simulink model "CompleteAttDetSim"  (R2018b)
settings: Solver=FixedStepAuto  StartTime=0.0  StopTime=24*3600  FixedStep=10  RelTol=1e-3  EnableMultiTasking=on
PreLoadFcn:
  | InitialiseJ2
values from neighbouring files (symbols this model uses):
  AngMomentum = (grav_parameter*rp*(1 + eccentricity))^0.5    [InitialiseJ2.m]
  Arg_periapsis = D3(1,6)    [InitialiseJ2.m]
  earthRadius = 6378.137    [InitialiseJ2.m]
  eccentricity = D3(1,5)/1e7    [InitialiseJ2.m]
  grav_parameter = 398600.4415    [InitialiseJ2.m]
  inclination = D3(1,3)    [InitialiseJ2.m]
  J2 = 0.0010836    [InitialiseJ2.m]
  period = 2*pi*sqrt(sm_axis^3/grav_parameter)    [InitialiseJ2.m]
  RAAN = D3(1,4)    [InitialiseJ2.m]
  sm_axis = (grav_parameter/(avg_motion*2*pi/(24*3600))^2)^(1/3)    [InitialiseJ2.m]
  t0 = avg_anomaly/(2*pi)*period    [InitialiseJ2.m]
undefined symbols (not defined in the file or in its folder): Earth, WGS84
libraries: vrlib x11, sharedtransform x7, simulink x6, aerolibutil x4, aerolibtransform2 x1
(part 1 of 2)
settings Model: PauseTimes=0  NumberOfSteps=10  SnapshotBufferSize=10000  SnapshotInterval=1  Creator="TEAM  STUDSAT -2"  LastModifiedBy=lauren
settings OptimizationCC: LifeSpan=inf
settings DebuggingCC: SFUnexpectedBacktrackingDiag=warning  SFNoUnconditionalDefaultTransitionDiag=warning  SFExecutionAtInitializationDiag=none
settings SFSimCC: SimUseLocalCustomCode=off
settings RTWCC: RTWUseLocalCustomCode=off
settings CodeAppCC: StateflowObjectComments=on
settings GRTTargetCC: TargetLangStandard=C89/C90 (ANSI)  GeneratePreprocessorConditionals=Disable all
settings ConfigComp: CovMetricSettings=dw  CovHtmlReporting=on  CovSaveCumulativeToWorkspaceVar=on  CovSaveSingleToWorkspaceVar=on  CovExternalEMLEnable=off
settings SimscapeCC: SimscapeNormalizeSystem=off

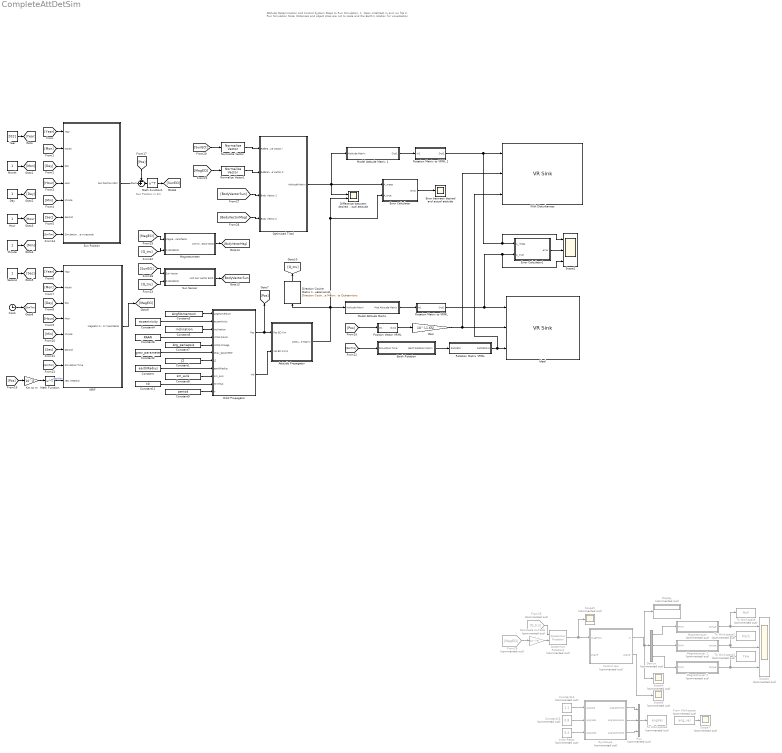
== system CompleteAttDetSim ==
  note: Sun Position in Km
  note: Attitude Determination and Control System
      |
      | Steps to Run Simulation:
      | 1. Open initalizeJ2.m and run file
      | 2. Run Simulation
      |
      | Note:
      | Distances and object sizes are not to scale and the Earth's rotation for visualisation
  " Magnetometer" : Subsystem
  " Sun Position" : Subsystem
  Attitude Propagator : Subsystem
  Clock : Clock
  Constant : Constant  Value=earthRadius
  Constant1 : Constant  Value=J2
  Constant11 : Constant  Value=t0
  Constant14 : Constant  Commented=on  Value=1.1
  Constant15 : Constant  Commented=on  Value=0.8
  Constant2 : Constant  Value=grav_parameter
  Constant3 : Constant  Value=AngMomentum
  Constant4 : Constant  Value=eccentricity
  Constant5 : Constant  Value=inclination
  Constant6 : Constant  Value=RAAN
  Constant7 : Constant  Value=Arg_periapsis
  Constant8 : Constant  Value=sm_axis
  Constant9 : Constant  Value=period
  Control Law : MATLAB Function  Commented=on  TreatAsAtomicUnit=on
  Day : Constant
  Demux : Demux  Commented=on  Outputs=3
  Difference between desired and actual attitude : Scope  NumInputPorts=2
  Direction Cosine Matrix to Quaternions1 : sharedtransform/Direction Cosine Matrix  to Quaternions  aMode=aMode  action=None  tolerance=eps(2)
      settings: SourceProductName=Aerospace Blockset  SourceProductBaseCode=AE
  Display : Display  Commented=on
  Earth Rotation : Subsystem
  Error Calculator : Subsystem
  Error Calculator1 : Subsystem
  Error between desired and actual attitude : Scope
  From Workspace : FromWorkspace  Commented=on  VariableName=ang_vel  SampleTime=0
  From28 : From  Commented=on  GotoTag=MagECI
  From29 : From  Commented=on  GotoTag=Q_tru
  Gain : Gain  Gain=10^(-1.65)
  Gyroscope : Subsystem  Commented=on
  Hour : Constant
  IGRF : Subsystem
  Ideal : vrlib/VR Sink  InstantiateOnLoad=on  SampleTime=-1  ViewEnable=on  RemoteChange=off  RemoteView=off  FieldsWritten=Satellite.rotation.4.1.1.double#Satellite.translation.3.1.1.double#Earth.rotation.4.1.1.double  WorldFileName=earthSatSys_Ideal.WRL  AutoView=off  VideoDimensions=[]  AllowVariableSize=off
      settings: SourceProductBaseCode=VR
  "Initial Rates " : Constant  Commented=on  Value=0.4
  Km to m : Gain  Gain=10^3
  "Magnetorquer " : Subsystem  Commented=on
  Magnetorquer 1 : Subsystem  Commented=on
  Magnetorquer 2 : Subsystem  Commented=on
  Math Function : Math  Operator=transpose  SaturateOnIntegerOverflow=on
  Math Function1 : Math  Operator=transpose  SaturateOnIntegerOverflow=on
  Minute : Constant
  Model Attitude Martix : Subsystem
  Model Attitude Matrix 1 : Subsystem
  Month : Constant
  Mux : Mux  Commented=on  Inputs=3
  Nanotesla to Tesla : Gain  Commented=on  Gain=10^(-9)
  Normalize Vector : vrlib/Utilities/Normalize Vector  maxzero=0
      settings: SourceProductName=Simulink 3D Animation  SourceProductBaseCode=VR
  Normalize Vector1 : vrlib/Utilities/Normalize Vector  maxzero=0
      settings: SourceProductName=Simulink 3D Animation  SourceProductBaseCode=VR
  Optimised Triad : Subsystem
  Orbit Propagator : Subsystem
  Position Vector VRML : Subsystem
  Quaternion Rotation1 : aerolibutil/Quaternion Rotation  Commented=on
  Rotation Matrix VRML : Subsystem
  "Rotation Matrix to VRML " : Subsystem
  Rotation Matrix to VRML 1 : Subsystem
  Scope1 : Scope  NumInputPorts=3
  Scope2 : Scope  Commented=on  NumInputPorts=3
  Scope{4..7} (4 alike) : Scope  Commented=on
  Second : Constant
  Sum : Sum  Inputs=-+|
  Sun Sensor : Subsystem
  To Workspace : ToWorkspace  Commented=on  VariableName=Roll  SampleTime=-1
  To Workspace1 : ToWorkspace  Commented=on  VariableName=Yaw  SampleTime=-1
  To Workspace2 : ToWorkspace  Commented=on  VariableName=Pitch  SampleTime=-1
  To Workspace3 : ToWorkspace  Commented=on  VariableName=angVel  SaveFormat=Timeseries  SampleTime=-1
  With Disturbances : vrlib/VR Sink  InstantiateOnLoad=on  SampleTime=-1  ViewEnable=on  RemoteChange=off  RemoteView=off  FieldsWritten=Satellite1.rotation.4.1.1.double#Satellite1.translation.3.1.1.double#Earth1.rotation.4.1.1.double  WorldFileName=earthSatSys_Real.WRL  AutoView=off  VideoDimensions=[]  AllowVariableSize=off
      settings: SourceProductBaseCode=VR
  Year : Constant  Value=2021
  wires:
  Constant/1 -> Orbit Propagator/8(earthRadius)
  Constant1/1 -> Orbit Propagator/7(J2)
  Constant2/1 -> Orbit Propagator/6(Grav_parameter)
  Constant3/1 -> Orbit Propagator/1(angMomentum)
  Constant4/1 -> Orbit Propagator/2(eccentricity)
  Constant5/1 -> Orbit Propagator/3(inclination)
  Constant6/1 -> Orbit Propagator/4(initial RAAN)
  Constant8/1 -> Orbit Propagator/9(sm_axis)
  Constant11/1 -> Orbit Propagator/10(t0 initial)
  Constant9/1 -> Orbit Propagator/11(T)
  Constant7/1 -> Orbit Propagator/5(initial Omega)
  Earth Rotation/1(Earth Rotation Matrix) -> Rotation Matrix VRML/1(RotMatIn)
  Position Vector VRML/1(Out1) -> Gain/1
  Gain/1 -> With Disturbances/2, Ideal/2
  Model Attitude Martix/1(Mod Attitude Matrix) -> "Rotation Matrix to VRML "/1(In1)
  Orbit Propagator/2(Vel) -> Attitude Propagator/2(Vel ECI Km/s)
  "Rotation Matrix to VRML "/1(Out1) -> Ideal/1, Scope1/3, Error Calculator1/2(A_true)
  Model Attitude Matrix 1/1(Out1) -> Rotation Matrix to VRML 1/1(In1)
  Rotation Matrix to VRML 1/1(Out1) -> Scope1/1, Error Calculator1/1(A_meas), With Disturbances/1
  Km to m/1 -> Math Function/1
  " Sun Position"/1(Sun Position (ECI)) -> Sum/2
  Year/1 -> [Year]
  Month/1 -> [Mon]
  Day/1 -> [Day]
  Hour/1 -> [Hour]
  Minute/1 -> [Min]
  Second/1 -> [Sec]
  [Year] -> " Sun Position"/1(Year)
  [Mon] -> " Sun Position"/2("Month ")
  [Day] -> " Sun Position"/3(Day)
  [Hour] -> " Sun Position"/4(Hour)
  [Min] -> " Sun Position"/5(Minute)
  [Sec] -> " Sun Position"/6(Second)
  [Year] -> IGRF/1(Year)
  [Mon] -> IGRF/2(Month)
  [Day] -> IGRF/3(Day)
  [Hour] -> IGRF/4(Hour)
  [Min] -> IGRF/5(Minute)
  [Sec] -> IGRF/6(Second)
  Clock/1 -> [SimTim]
  [SimTim] -> Earth Rotation/1(Simulation Time)
  [SimTim] -> IGRF/7(Simulation Time)
  [SimTim] -> " Sun Position"/7(Simulation time in seconds)
  Orbit Propagator/1(Pos) -> Attitude Propagator/1(Pos ECI Km), [Pos]
  [Pos] -> Position Vector VRML/1(In1)
  [Pos] -> Km to m/1
  Math Function/1 -> IGRF/8(rECI (Meters))  "position"
  [Pos] -> Sum/1
  Sum/1 -> Math Function1/1
  IGRF/1(Magnetic Field in ECI (nanoTesla)) -> [MagECI]
  [SunECI] -> Sun Sensor/1(Sun Vector)
  [MagECI] -> " Magnetometer"/1(Magnettic Field ECI nanoTesla)
  [SunECI] -> Normalize Vector/1
  [MagECI] -> Normalize Vector1/1
  Normalize Vector/1 -> Optimised Triad/1(Reference Vector !)
  Normalize Vector1/1 -> Optimised Triad/2(Reference Vector 2)
  Direction Cosine Matrix to Quaternions1/1 -> [Q_tru]
  [Q_tru] -> " Magnetometer"/2(Q ECI2BOD)
  [Q_tru] -> Sun Sensor/2(Q ECI2BOD)
  Math Function1/1 -> [SunECI]
  Optimised Triad/1(Attitude Matrix) -> Difference between desired and actual attitude/1, Error Calculator/1(A_meas), Model Attitude Matrix 1/1(Attitude Matrix)
  Attitude Propagator/1(Attitude Matrix) -> Model Attitude Martix/1(Attitude Matrix), Error Calculator/2(A_true), Difference between desired and actual attitude/2, Direction Cosine Matrix to Quaternions1/1
  Sun Sensor/1(Unit Sun Vector BOD) -> [BodyVectorSun]
  [BodyVectorSun] -> Optimised Triad/3(Body Vector 1)
  [BodyVectorMag] -> Optimised Triad/4(Body Vector 2)
  Error Calculator1/1(error) -> Scope1/2
  Error Calculator/1(error) -> Error between desired and actual attitude/1
  Rotation Matrix VRML/1(RotMatOut) -> With Disturbances/3, Ideal/3
  " Magnetometer"/1(Unit Magnetic Field Vector BOD) -> [BodyVectorMag]
  Gyroscope/1(angratenoise) -> Mux/1
  Gyroscope/2("angratenoise1 ") -> Mux/2
  Gyroscope/3("angratenoise2 ") -> Mux/3
  Demux/1 -> "Magnetorquer "/1(PWM)
  Demux/2 -> Magnetorquer 1/1("PWM ")
  Demux/3 -> Magnetorquer 2/1(PWM)
  Magnetorquer 1/1(torque) -> Scope2/2, To Workspace2/1
  "Magnetorquer "/1(torque) -> Scope2/1, To Workspace/1
  Magnetorquer 2/1(torque) -> Scope2/3, To Workspace1/1
  Control Law/1(m) -> Scope4/1, Display/1, Demux/1
  Nanotesla to Tesla/1 -> Quaternion Rotation1/2
  From28/1 -> Nanotesla to Tesla/1
  From29/1 -> Quaternion Rotation1/1
  Quaternion Rotation1/1 -> Scope5/1, Control Law/1(magField)
  Control Law/2(angvel) -> Scope6/1
  Constant14/1 -> Gyroscope/1(angrate)
  Constant15/1 -> Gyroscope/2("angrate1 ")
  "Initial Rates "/1 -> Gyroscope/3(angrate2)
  Mux/1 -> To Workspace3/1
  From Workspace/1 -> Scope7/1

== system CompleteAttDetSim/ Magnetometer ==
  Magnettic Field ECI nanoTesla : Inport
  Q ECI2BOD : Inport  Port=2
  Magnetometer Error : Subsystem
  Nanotesla to Tesla : Gain  Gain=10^(-9)
  Normalize Vector5 : vrlib/Utilities/Normalize Vector  maxzero=0
      settings: SourceProductName=Simulink 3D Animation  SourceProductBaseCode=VR
  Quaternion Rotation1 : aerolibutil/Quaternion Rotation
  Unit Magnetic Field Vector BOD : Outport
  wires:
  Magnettic Field ECI nanoTesla/1 -> Nanotesla to Tesla/1
  Magnetometer Error/1("Magnetic Field BOD (Tesla)1 ") -> Normalize Vector5/1
  Normalize Vector5/1 -> Unit Magnetic Field Vector BOD/1
  Q ECI2BOD/1 -> Quaternion Rotation1/1
  Nanotesla to Tesla/1 -> Quaternion Rotation1/2
  Quaternion Rotation1/1 -> Magnetometer Error/1(Magnetic Field BOD (Tesla))

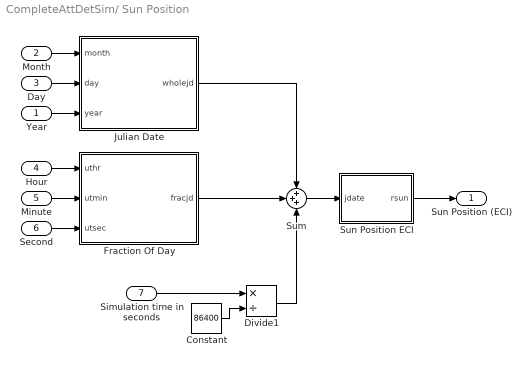
== system CompleteAttDetSim/ Sun Position ==
  Year : Inport
  "Month " : Inport  Port=2
  Day : Inport  Port=3
  Hour : Inport  Port=4
  Minute : Inport  Port=5
  Second : Inport  Port=6
  Simulation time in seconds : Inport  Port=7
  Constant : Constant  Value=86400
  Divide1 : Product  Inputs=*/
  Fraction Of Day : MATLAB Function  TreatAsAtomicUnit=on
  Julian Date : MATLAB Function  TreatAsAtomicUnit=on
  Sum : Sum  Inputs=+++
  Sun Position ECI : MATLAB Function  TreatAsAtomicUnit=on
  Sun Position (ECI) : Outport
  wires:
  Sum/1 -> Sun Position ECI/1(jdate)
  Simulation time in seconds/1 -> Divide1/1
  Sun Position ECI/1(rsun) -> Sun Position (ECI)/1
  Second/1 -> Fraction Of Day/3(utsec)
  Fraction Of Day/1(fracjd) -> Sum/2
  Year/1 -> Julian Date/3(year)
  Day/1 -> Julian Date/2(day)
  Divide1/1 -> Sum/3
  Minute/1 -> Fraction Of Day/2(utmin)
  Julian Date/1(wholejd) -> Sum/1
  Constant/1 -> Divide1/2
  Hour/1 -> Fraction Of Day/1(uthr)
  "Month "/1 -> Julian Date/1(month)

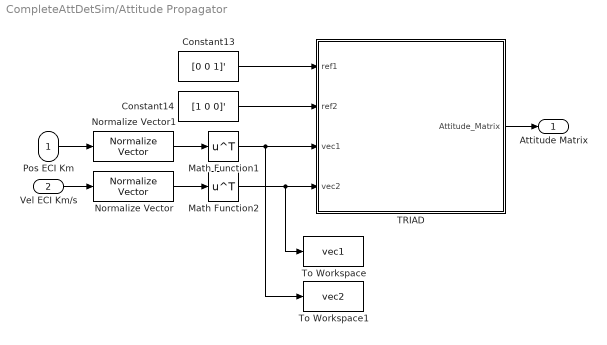
== system CompleteAttDetSim/Attitude Propagator ==
  Pos ECI Km : Inport
  Vel ECI Km/s : Inport  Port=2
  Constant13 : Constant  Value=[0 0 1]'  VectorParams1D=off
  Constant14 : Constant  Value=[1 0 0]'  VectorParams1D=off
  Math Function1 : Math  Operator=transpose  SaturateOnIntegerOverflow=on
  Math Function2 : Math  Operator=transpose  SaturateOnIntegerOverflow=on
  Normalize Vector : vrlib/Utilities/Normalize Vector  maxzero=0
      settings: SourceProductName=Simulink 3D Animation  SourceProductBaseCode=VR
  Normalize Vector1 : vrlib/Utilities/Normalize Vector  maxzero=0
      settings: SourceProductName=Simulink 3D Animation  SourceProductBaseCode=VR
  TRIAD : MATLAB Function  TreatAsAtomicUnit=on
  To Workspace : ToWorkspace  VariableName=vec1  SampleTime=-1
  To Workspace1 : ToWorkspace  VariableName=vec2  SampleTime=-1
  Attitude Matrix : Outport
  wires:
  Constant13/1 -> TRIAD/1(ref1)
  TRIAD/1(Attitude_Matrix) -> Attitude Matrix/1
  Math Function1/1 -> To Workspace1/1, TRIAD/3(vec1)
  Math Function2/1 -> To Workspace/1, TRIAD/4(vec2)
  Constant14/1 -> TRIAD/2(ref2)
  Vel ECI Km/s/1 -> Normalize Vector/1
  Normalize Vector/1 -> Math Function2/1
  Normalize Vector1/1 -> Math Function1/1
  Pos ECI Km/1 -> Normalize Vector1/1

== system CompleteAttDetSim/Earth Rotation ==
  Simulation Time : Inport
  Constant10 : Constant  Value=0.004178074378280
  Subsystem1 : Subsystem
  Earth Rotation Matrix : Outport
  wires:
  Constant10/1 -> Subsystem1/1(we)
  Simulation Time/1 -> Subsystem1/2(Clock)
  Subsystem1/1(Earth Rotation Matrix) -> Earth Rotation Matrix/1

== system CompleteAttDetSim/Error Calculator ==
  A_meas : Inport
  A_true : Inport  Port=2
  Subtract : Sum  Inputs=+-
  error : Outport
  wires:
  Subtract/1 -> error/1
  A_meas/1 -> Subtract/1
  A_true/1 -> Subtract/2

== system CompleteAttDetSim/Error Calculator1 ==
  A_meas : Inport
  A_true : Inport  Port=2
  Subtract : Sum  Inputs=+-
  error : Outport
  wires:
  Subtract/1 -> error/1
  A_meas/1 -> Subtract/1
  A_true/1 -> Subtract/2

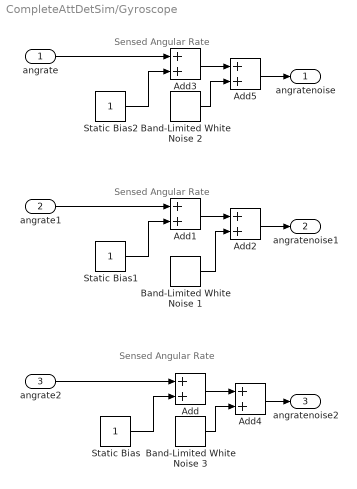
== system CompleteAttDetSim/Gyroscope ==
  note: Sensed Angular Rate
  note: Sensed Angular Rate
  note: Sensed Angular Rate
  angrate : Inport
  "angrate1 " : Inport  Port=2
  angrate2 : Inport  Port=3
  Add{,1..5} (6 alike) : Sum
  Band-Limited White Noise 1 : simulink/Sources/Band-Limited White Noise  Cov=[0.018^2]  Ts=10  seed=[23341]
  Band-Limited White Noise 2 : simulink/Sources/Band-Limited White Noise  Cov=[0.018^2]  Ts=10  seed=[23341]
  Band-Limited White Noise 3 : simulink/Sources/Band-Limited White Noise  Cov=[0.018^2]  Ts=10  seed=[23341]
  Static Bias : Constant
  Static Bias1 : Constant
  Static Bias2 : Constant
  angratenoise : Outport
  "angratenoise1 " : Outport  Port=2
  "angratenoise2 " : Outport  Port=3
  wires:
  Add4/1 -> "angratenoise2 "/1
  Add2/1 -> "angratenoise1 "/1
  Add5/1 -> angratenoise/1
  Band-Limited White Noise 3/1 -> Add4/2
  Static Bias/1 -> Add/2
  Add/1 -> Add4/1
  angrate2/1 -> Add/1
  Static Bias1/1 -> Add1/2
  Add1/1 -> Add2/1
  Band-Limited White Noise 1/1 -> Add2/2
  "angrate1 "/1 -> Add1/1
  Static Bias2/1 -> Add3/2
  Add3/1 -> Add5/1
  Band-Limited White Noise 2/1 -> Add5/2
  angrate/1 -> Add3/1

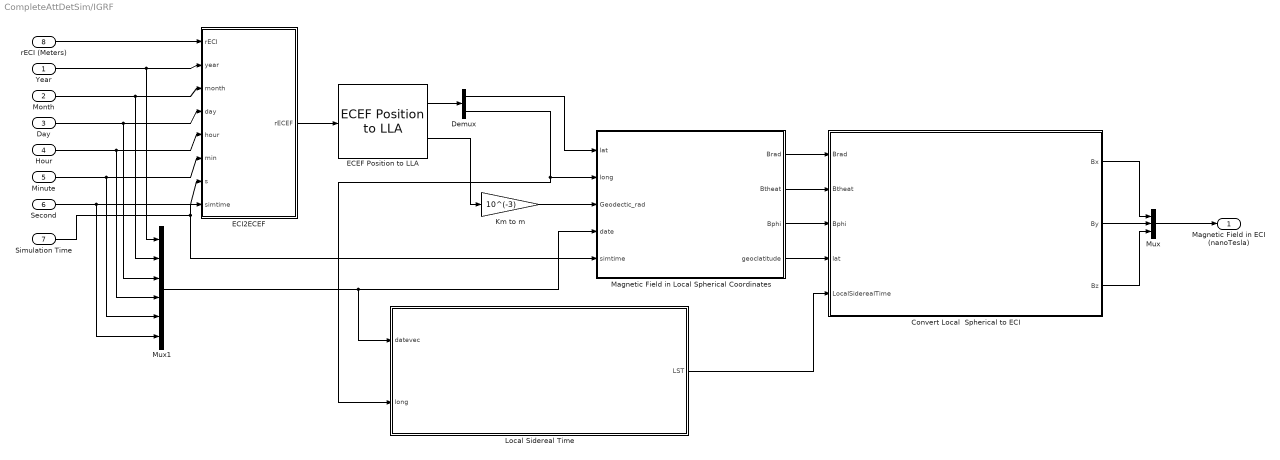
== system CompleteAttDetSim/IGRF ==
  Year : Inport
  Month : Inport  Port=2
  Day : Inport  Port=3
  Hour : Inport  Port=4
  Minute : Inport  Port=5
  Second : Inport  Port=6
  Simulation Time : Inport  Port=7
  rECI (Meters) : Inport  Port=8
  Convert Local  Spherical to ECI : MATLAB Function  TreatAsAtomicUnit=on
  Demux : Demux  Outputs=2
  ECEF Position to LLA : aerolibtransform2/ECEF Position to LLA  units=Metric (MKS)  ptype=Earth (WGS84)  F=1/298.257223563  R=6378137
      settings: SourceProductName=Aerospace Blockset  SourceProductBaseCode=AE
  ECI2ECEF : MATLAB Function  TreatAsAtomicUnit=on
  Km to m : Gain  Gain=10^(-3)
  Local Sidereal Time : MATLAB Function  TreatAsAtomicUnit=on
  Magnetic Field in Local Spherical Coordinates : MATLAB Function  TreatAsAtomicUnit=on
  Mux : Mux  Inputs=3
  Mux1 : Mux  Inputs=6
  Magnetic Field in ECI (nanoTesla) : Outport
  wires:
  Magnetic Field in Local Spherical Coordinates/2(Btheat) -> Convert Local  Spherical to ECI/2(Btheat)
  Day/1 -> Mux1/3, ECI2ECEF/4(day)
  Second/1 -> Mux1/6, ECI2ECEF/7(s)
  ECEF Position to LLA/1 -> Demux/1
  Convert Local  Spherical to ECI/3(Bz) -> Mux/3
  Magnetic Field in Local Spherical Coordinates/3(Bphi) -> Convert Local  Spherical to ECI/3(Bphi)
  Local Sidereal Time/1(LST) -> Convert Local  Spherical to ECI/5(LocalSiderealTime)
  Magnetic Field in Local Spherical Coordinates/1(Brad) -> Convert Local  Spherical to ECI/1(Brad)
  ECEF Position to LLA/2 -> Km to m/1
  Minute/1 -> Mux1/5, ECI2ECEF/6(min)
  ECI2ECEF/1(rECEF) -> ECEF Position to LLA/1
  Demux/1 -> Magnetic Field in Local Spherical Coordinates/1(lat)
  Month/1 -> Mux1/2, ECI2ECEF/3(month)
  Year/1 -> Mux1/1, ECI2ECEF/2(year)
  rECI (Meters)/1 -> ECI2ECEF/1(rECI)
  Convert Local  Spherical to ECI/1(Bx) -> Mux/1
  Magnetic Field in Local Spherical Coordinates/4(geoclatitude) -> Convert Local  Spherical to ECI/4(lat)
  Hour/1 -> Mux1/4, ECI2ECEF/5(hour)
  Mux1/1 -> Magnetic Field in Local Spherical Coordinates/4(date), Local Sidereal Time/1(datevec)
  Convert Local  Spherical to ECI/2(By) -> Mux/2
  Demux/2 -> Local Sidereal Time/2(long), Magnetic Field in Local Spherical Coordinates/2(long)
  Mux/1 -> Magnetic Field in ECI (nanoTesla)/1
  Simulation Time/1 -> ECI2ECEF/8(simtime), Magnetic Field in Local Spherical Coordinates/5(simtime)
  Km to m/1 -> Magnetic Field in Local Spherical Coordinates/3(Geodectic_rad)

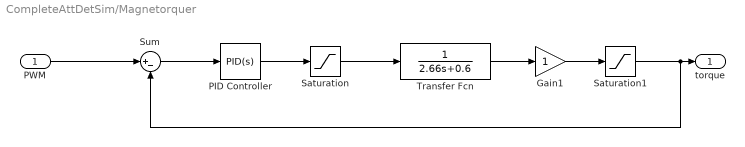
== system CompleteAttDetSim/Magnetorquer  ==
  PWM : Inport
  Gain1 : Gain
  PID Controller : simulink/Continuous/PID Controller  Controller=PID  Form=Parallel  TimeDomain=Continuous-time  SampleTime=-1  IntegratorMethod=Forward Euler  FilterMethod=Forward Euler  ControllerParametersSource=internal  P=3  I=1  D=0  UseFilter=on  N=100  TunerSelectOption=Transfer Function Based (PID Tuner App)  InitialConditionSource=internal  InitialConditionForIntegrator=0  InitialConditionForFilter=0  DifferentiatorICPrevScaledInput=0  ExternalReset=none  TrackingMode=off  Kt=1  LimitOutput=off  UpperSaturationLimit=inf  LowerSaturationLimit=-inf  LinearizeAsGain=on  AntiWindupMode=none  Kb=1  POutMin=[]  POutMax=[]  IOutMin=[]  IOutMax=[]  DOutMin=[]  DOutMax=[]  NOutMin=[]  NOutMax=[]  SumOutMin=[]  SumOutMax=[]  SaturationOutMin=[]  SaturationOutMax=[]  PParamMin=[]  PParamMax=[]  IParamMin=[]  IParamMax=[]  DParamMin=[]  DParamMax=[]  NParamMin=[]  NParamMax=[]  KbParamMin=[]  KbParamMax=[]  KtParamMin=[]  KtParamMax=[]  KbOutMin=[]  KbOutMax=[]  KtOutMin=[]  KtOutMax=[]  IntegratorOutMin=[]  IntegratorOutMax=[]  FilterOutMin=[]  FilterOutMax=[]  SumI1OutMin=[]  SumI1OutMax=[]  SumI2OutMin=[]  SumI2OutMax=[]  SumI3OutMin=[]  SumI3OutMax=[]  SumI4OutMin=[]  SumI4OutMax=[]  SumDOutMin=[]  SumDOutMax=[]  DifferentiatorOutMin=[]  DifferentiatorOutMax=[]  FilterDiffOutCoefMin=[]  FilterDiffOutCoefMax=[]  ReciprocalOutMin=[]  ReciprocalOutMax=[]  SumDenOutMin=[]  SumDenOutMax=[]  SumNumOutMin=[]  SumNumOutMax=[]  DivideOutMin=[]  DivideOutMax=[]  IntegratorContinuousStateAttributes=''  IntegratorStateMustResolveToSignalObject=off  IntegratorRTWStateStorageClass=Auto  FilterContinuousStateAttributes=''  FilterStateMustResolveToSignalObject=off  FilterRTWStateStorageClass=Auto  ParallelPVariant=InternalParameters  IdealPVariant=Disabled  IVariant=InternalParameters  DVariant=InternalParameters  IntegratorVariant=Continuous  SatVariant=Disabled  AWVariant=Passthrough  PCopyVariant=Disabled  TRVariant=Disabled  FdbkBlocksVariant=Forward  IdealPFdbkVariant=Disabled  SatFdbkVariant=Disabled  DerivativeFilterVariant=ContFilter  NVariant=InternalParameters  NCopyVariant=Disabled  FilterICVariant=InternalICsFilter  IntegratorICVariant=InternalICs  ExternalResetVariant=Disabled  TRSumVariant=Passthrough  SumFdbkVariant=Disabled  SumVariant=Sum_PID
  Saturation : Saturate
  Saturation1 : Saturate
  Sum : Sum  Inputs=|+-
  Transfer Fcn : TransferFcn  Denominator=[2.66 0.6]
  torque : Outport
  wires:
  Gain1/1 -> Saturation1/1
  PID Controller/1 -> Saturation/1
  Transfer Fcn/1 -> Gain1/1
  PWM/1 -> Sum/1
  Sum/1 -> PID Controller/1
  Saturation/1 -> Transfer Fcn/1
  Saturation1/1 -> Sum/2, torque/1

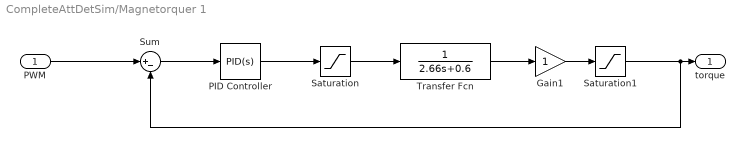
== system CompleteAttDetSim/Magnetorquer 1 ==
  "PWM " : Inport
  Gain1 : Gain
  PID Controller : simulink/Continuous/PID Controller  Controller=PID  Form=Parallel  TimeDomain=Continuous-time  SampleTime=-1  IntegratorMethod=Forward Euler  FilterMethod=Forward Euler  ControllerParametersSource=internal  P=3  I=1  D=0  UseFilter=on  N=100  TunerSelectOption=Transfer Function Based (PID Tuner App)  InitialConditionSource=internal  InitialConditionForIntegrator=0  InitialConditionForFilter=0  DifferentiatorICPrevScaledInput=0  ExternalReset=none  TrackingMode=off  Kt=1  LimitOutput=off  UpperSaturationLimit=inf  LowerSaturationLimit=-inf  LinearizeAsGain=on  AntiWindupMode=none  Kb=1  POutMin=[]  POutMax=[]  IOutMin=[]  IOutMax=[]  DOutMin=[]  DOutMax=[]  NOutMin=[]  NOutMax=[]  SumOutMin=[]  SumOutMax=[]  SaturationOutMin=[]  SaturationOutMax=[]  PParamMin=[]  PParamMax=[]  IParamMin=[]  IParamMax=[]  DParamMin=[]  DParamMax=[]  NParamMin=[]  NParamMax=[]  KbParamMin=[]  KbParamMax=[]  KtParamMin=[]  KtParamMax=[]  KbOutMin=[]  KbOutMax=[]  KtOutMin=[]  KtOutMax=[]  IntegratorOutMin=[]  IntegratorOutMax=[]  FilterOutMin=[]  FilterOutMax=[]  SumI1OutMin=[]  SumI1OutMax=[]  SumI2OutMin=[]  SumI2OutMax=[]  SumI3OutMin=[]  SumI3OutMax=[]  SumI4OutMin=[]  SumI4OutMax=[]  SumDOutMin=[]  SumDOutMax=[]  DifferentiatorOutMin=[]  DifferentiatorOutMax=[]  FilterDiffOutCoefMin=[]  FilterDiffOutCoefMax=[]  ReciprocalOutMin=[]  ReciprocalOutMax=[]  SumDenOutMin=[]  SumDenOutMax=[]  SumNumOutMin=[]  SumNumOutMax=[]  DivideOutMin=[]  DivideOutMax=[]  IntegratorContinuousStateAttributes=''  IntegratorStateMustResolveToSignalObject=off  IntegratorRTWStateStorageClass=Auto  FilterContinuousStateAttributes=''  FilterStateMustResolveToSignalObject=off  FilterRTWStateStorageClass=Auto  ParallelPVariant=InternalParameters  IdealPVariant=Disabled  IVariant=InternalParameters  DVariant=InternalParameters  IntegratorVariant=Continuous  SatVariant=Disabled  AWVariant=Passthrough  PCopyVariant=Disabled  TRVariant=Disabled  FdbkBlocksVariant=Forward  IdealPFdbkVariant=Disabled  SatFdbkVariant=Disabled  DerivativeFilterVariant=ContFilter  NVariant=InternalParameters  NCopyVariant=Disabled  FilterICVariant=InternalICsFilter  IntegratorICVariant=InternalICs  ExternalResetVariant=Disabled  TRSumVariant=Passthrough  SumFdbkVariant=Disabled  SumVariant=Sum_PID
  Saturation : Saturate
  Saturation1 : Saturate
  Sum : Sum  Inputs=|+-
  Transfer Fcn : TransferFcn  Denominator=[2.66 0.6]
  torque : Outport
  wires:
  Gain1/1 -> Saturation1/1
  PID Controller/1 -> Saturation/1
  Transfer Fcn/1 -> Gain1/1
  "PWM "/1 -> Sum/1
  Sum/1 -> PID Controller/1
  Saturation/1 -> Transfer Fcn/1
  Saturation1/1 -> Sum/2, torque/1

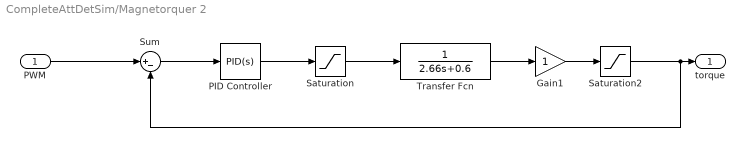
== system CompleteAttDetSim/Magnetorquer 2 ==
  PWM : Inport
  Gain1 : Gain
  PID Controller : simulink/Continuous/PID Controller  Controller=PID  Form=Parallel  TimeDomain=Continuous-time  SampleTime=-1  IntegratorMethod=Forward Euler  FilterMethod=Forward Euler  ControllerParametersSource=internal  P=3  I=1  D=0  UseFilter=on  N=100  TunerSelectOption=Transfer Function Based (PID Tuner App)  InitialConditionSource=internal  InitialConditionForIntegrator=0  InitialConditionForFilter=0  DifferentiatorICPrevScaledInput=0  ExternalReset=none  TrackingMode=off  Kt=1  LimitOutput=off  UpperSaturationLimit=inf  LowerSaturationLimit=-inf  LinearizeAsGain=on  AntiWindupMode=none  Kb=1  POutMin=[]  POutMax=[]  IOutMin=[]  IOutMax=[]  DOutMin=[]  DOutMax=[]  NOutMin=[]  NOutMax=[]  SumOutMin=[]  SumOutMax=[]  SaturationOutMin=[]  SaturationOutMax=[]  PParamMin=[]  PParamMax=[]  IParamMin=[]  IParamMax=[]  DParamMin=[]  DParamMax=[]  NParamMin=[]  NParamMax=[]  KbParamMin=[]  KbParamMax=[]  KtParamMin=[]  KtParamMax=[]  KbOutMin=[]  KbOutMax=[]  KtOutMin=[]  KtOutMax=[]  IntegratorOutMin=[]  IntegratorOutMax=[]  FilterOutMin=[]  FilterOutMax=[]  SumI1OutMin=[]  SumI1OutMax=[]  SumI2OutMin=[]  SumI2OutMax=[]  SumI3OutMin=[]  SumI3OutMax=[]  SumI4OutMin=[]  SumI4OutMax=[]  SumDOutMin=[]  SumDOutMax=[]  DifferentiatorOutMin=[]  DifferentiatorOutMax=[]  FilterDiffOutCoefMin=[]  FilterDiffOutCoefMax=[]  ReciprocalOutMin=[]  ReciprocalOutMax=[]  SumDenOutMin=[]  SumDenOutMax=[]  SumNumOutMin=[]  SumNumOutMax=[]  DivideOutMin=[]  DivideOutMax=[]  IntegratorContinuousStateAttributes=''  IntegratorStateMustResolveToSignalObject=off  IntegratorRTWStateStorageClass=Auto  FilterContinuousStateAttributes=''  FilterStateMustResolveToSignalObject=off  FilterRTWStateStorageClass=Auto  ParallelPVariant=InternalParameters  IdealPVariant=Disabled  IVariant=InternalParameters  DVariant=InternalParameters  IntegratorVariant=Continuous  SatVariant=Disabled  AWVariant=Passthrough  PCopyVariant=Disabled  TRVariant=Disabled  FdbkBlocksVariant=Forward  IdealPFdbkVariant=Disabled  SatFdbkVariant=Disabled  DerivativeFilterVariant=ContFilter  NVariant=InternalParameters  NCopyVariant=Disabled  FilterICVariant=InternalICsFilter  IntegratorICVariant=InternalICs  ExternalResetVariant=Disabled  TRSumVariant=Passthrough  SumFdbkVariant=Disabled  SumVariant=Sum_PID
  Saturation : Saturate
  Saturation2 : Saturate
  Sum : Sum  Inputs=|+-
  Transfer Fcn : TransferFcn  Denominator=[2.66 0.6]
  torque : Outport
  wires:
  Gain1/1 -> Saturation2/1
  PID Controller/1 -> Saturation/1
  Transfer Fcn/1 -> Gain1/1
  PWM/1 -> Sum/1
  Sum/1 -> PID Controller/1
  Saturation/1 -> Transfer Fcn/1
  Saturation2/1 -> Sum/2, torque/1

== system CompleteAttDetSim/Model Attitude Martix ==
  Attitude Matrix : Inport
  Constant10 : Constant  Value=-90
  Matrix Multiply1 : Product  Multiplication=Matrix(*)
  Rotate about x1 : MATLAB Function  TreatAsAtomicUnit=on
  Mod Attitude Matrix : Outport
  wires:
  Constant10/1 -> Rotate about x1/1(u)
  Matrix Multiply1/1 -> Mod Attitude Matrix/1
  Attitude Matrix/1 -> Matrix Multiply1/1
  Rotate about x1/1(y) -> Matrix Multiply1/2

== system CompleteAttDetSim/Model Attitude Matrix 1 ==
  Attitude Matrix : Inport
  Constant10 : Constant  Value=-90
  Matrix Multiply1 : Product  Multiplication=Matrix(*)
  Rotate about x1 : MATLAB Function  TreatAsAtomicUnit=on
  Out1 : Outport
  wires:
  Constant10/1 -> Rotate about x1/1(u)
  Matrix Multiply1/1 -> Out1/1
  Attitude Matrix/1 -> Matrix Multiply1/1
  Rotate about x1/1(y) -> Matrix Multiply1/2

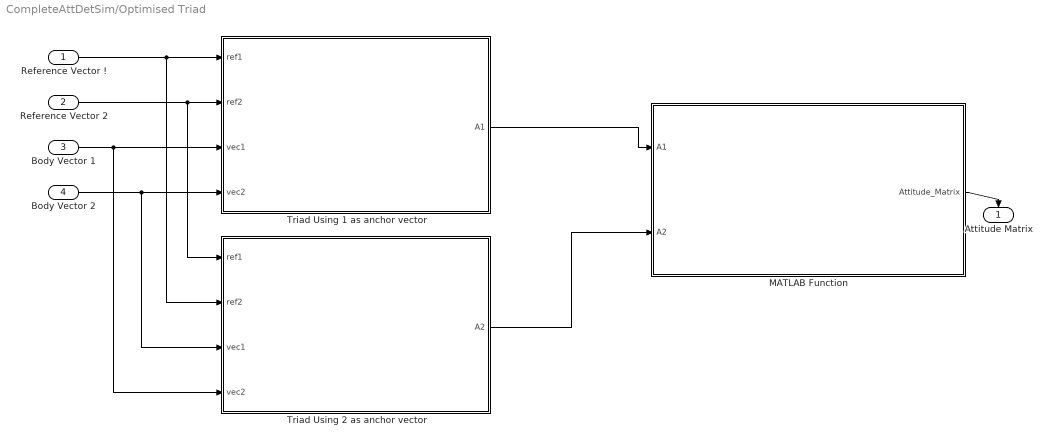
== system CompleteAttDetSim/Optimised Triad ==
  Reference Vector ! : Inport
  Reference Vector 2 : Inport  Port=2
  Body Vector 1 : Inport  Port=3
  Body Vector 2 : Inport  Port=4
  MATLAB Function : MATLAB Function  TreatAsAtomicUnit=on
  Triad Using 1 as anchor vector : MATLAB Function  TreatAsAtomicUnit=on
  Triad Using 2 as anchor vector : MATLAB Function  TreatAsAtomicUnit=on
  Attitude Matrix : Outport
  wires:
  Triad Using 1 as anchor vector/1(A1) -> MATLAB Function/1(A1)
  Body Vector 2/1 -> Triad Using 1 as anchor vector/4(vec2), Triad Using 2 as anchor vector/3(vec1)
  Body Vector 1/1 -> Triad Using 2 as anchor vector/4(vec2), Triad Using 1 as anchor vector/3(vec1)
  Triad Using 2 as anchor vector/1(A2) -> MATLAB Function/2(A2)
  Reference Vector 2/1 -> Triad Using 1 as anchor vector/2(ref2), Triad Using 2 as anchor vector/1(ref1)
  MATLAB Function/1(Attitude_Matrix) -> Attitude Matrix/1
  Reference Vector !/1 -> Triad Using 2 as anchor vector/2(ref2), Triad Using 1 as anchor vector/1(ref1)

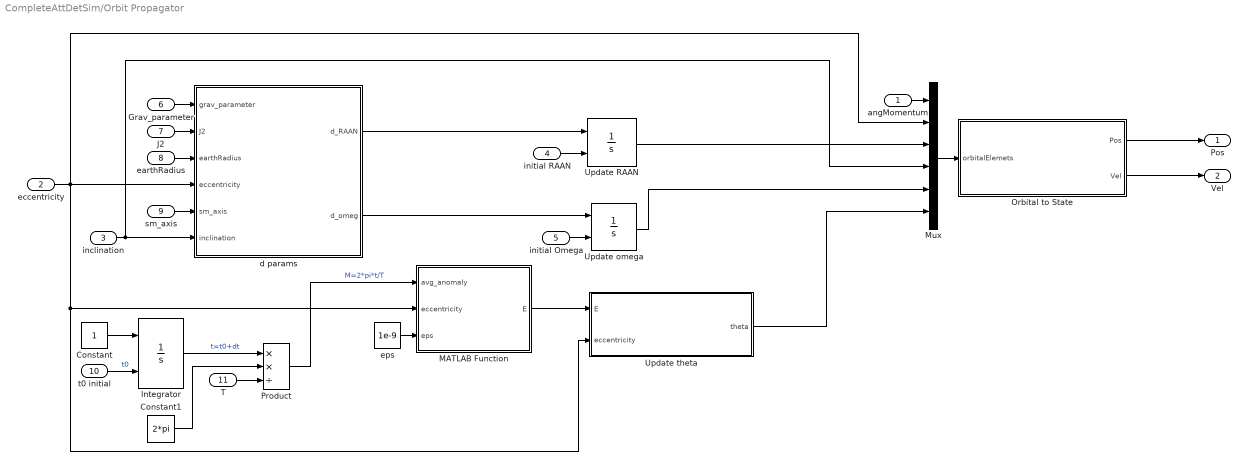
== system CompleteAttDetSim/Orbit Propagator ==
  angMomentum : Inport
  eccentricity : Inport  Port=2
  inclination : Inport  Port=3
  initial RAAN : Inport  Port=4
  initial Omega : Inport  Port=5
  Grav_parameter : Inport  Port=6
  J2 : Inport  Port=7
  earthRadius : Inport  Port=8
  sm_axis : Inport  Port=9
  t0 initial : Inport  Port=10
  T : Inport  Port=11
  Constant : Constant
  Constant1 : Constant  Value=2*pi
  Integrator : Integrator  InitialConditionSource=external
  MATLAB Function : MATLAB Function  TreatAsAtomicUnit=on
  Mux : Mux  Inputs=6
  Orbital to State : MATLAB Function  TreatAsAtomicUnit=on
  Product : Product  Inputs=**/
  Update RAAN : Integrator  InitialConditionSource=external
  Update omega : Integrator  InitialConditionSource=external
  Update theta : MATLAB Function  TreatAsAtomicUnit=on
  d params : MATLAB Function  TreatAsAtomicUnit=on
  eps : Constant  Value=1e-9
  Pos : Outport
  Vel : Outport  Port=2
  wires:
  eps/1 -> MATLAB Function/3(eps)
  Grav_parameter/1 -> d params/1(grav_parameter)
  sm_axis/1 -> d params/5(sm_axis)
  J2/1 -> d params/2(J2)
  earthRadius/1 -> d params/3(earthRadius)
  MATLAB Function/1(E) -> Update theta/1(E)
  t0 initial/1 -> Integrator/2  "t0"
  Constant/1 -> Integrator/1
  Integrator/1 -> Product/1  "t=t0+dt"
  T/1 -> Product/3
  Constant1/1 -> Product/2
  d params/1(d_RAAN) -> Update RAAN/1
  initial RAAN/1 -> Update RAAN/2
  d params/2(d_omeg) -> Update omega/1
  initial Omega/1 -> Update omega/2
  angMomentum/1 -> Mux/1
  inclination/1 -> Mux/4, d params/6(inclination)
  Mux/1 -> Orbital to State/1(orbitalElemets)
  Product/1 -> MATLAB Function/1(avg_anomaly)  "M=2*pi*t/T"
  Update omega/1 -> Mux/5
  Update theta/1(theta) -> Mux/6
  Update RAAN/1 -> Mux/3
  eccentricity/1 -> Update theta/2(eccentricity), MATLAB Function/2(eccentricity), Mux/2, d params/4(eccentricity)
  Orbital to State/1(Pos) -> Pos/1
  Orbital to State/2(Vel) -> Vel/1

== system CompleteAttDetSim/Position Vector VRML ==
  In1 : Inport
  Demux : Demux  Outputs=3
  Gain2 : Gain  Gain=-1
  Mux : Mux  Inputs=3
  Out1 : Outport
  wires:
  Demux/1 -> Mux/1
  Demux/2 -> Gain2/1
  Demux/3 -> Mux/2
  Mux/1 -> Out1/1
  Gain2/1 -> Mux/3
  In1/1 -> Demux/1

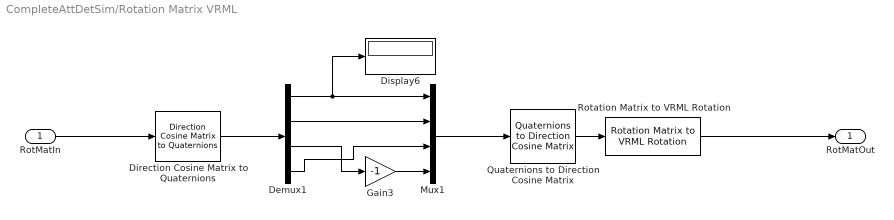
== system CompleteAttDetSim/Rotation Matrix VRML ==
  RotMatIn : Inport
  Demux1 : Demux
  Direction Cosine Matrix to Quaternions : sharedtransform/Direction Cosine Matrix  to Quaternions  aMode=aMode  action=None  tolerance=eps(2)
      settings: SourceProductName=Aerospace Blockset  SourceProductBaseCode=AE
  Display6 : Display
  Gain3 : Gain  Gain=-1
  Mux1 : Mux
  Quaternions to Direction Cosine Matrix : sharedtransform/Quaternions to  Direction Cosine Matrix  aMode=aMode
      settings: SourceProductName=Aerospace Blockset  SourceProductBaseCode=AE
  Rotation Matrix to VRML Rotation : vrlib/Utilities/Rotation Matrix to VRML Rotation  maxzero=1e-12
      settings: SourceProductName=Simulink 3D Animation  SourceProductBaseCode=VR
  RotMatOut : Outport
  wires:
  RotMatIn/1 -> Direction Cosine Matrix to Quaternions/1
  Direction Cosine Matrix to Quaternions/1 -> Demux1/1
  Demux1/3 -> Gain3/1
  Gain3/1 -> Mux1/4
  Demux1/4 -> Mux1/3
  Demux1/2 -> Mux1/2
  Demux1/1 -> Display6/1, Mux1/1
  Mux1/1 -> Quaternions to Direction Cosine Matrix/1
  Quaternions to Direction Cosine Matrix/1 -> Rotation Matrix to VRML Rotation/1
  Rotation Matrix to VRML Rotation/1 -> RotMatOut/1

== system CompleteAttDetSim/Rotation Matrix to VRML  ==
  In1 : Inport
  Demux2 : Demux
  Direction Cosine Matrix to Quaternions1 : sharedtransform/Direction Cosine Matrix  to Quaternions  aMode=aMode  action=None  tolerance=eps(2)
      settings: SourceProductName=Aerospace Blockset  SourceProductBaseCode=AE
  Gain4 : Gain  Gain=-1
  Mux2 : Mux
  Quaternions to Direction Cosine Matrix1 : sharedtransform/Quaternions to  Direction Cosine Matrix  aMode=aMode
      settings: SourceProductName=Aerospace Blockset  SourceProductBaseCode=AE
  Rotation Matrix to VRML Rotation1 : vrlib/Utilities/Rotation Matrix to VRML Rotation  maxzero=1e-12
      settings: SourceProductName=Simulink 3D Animation  SourceProductBaseCode=VR
  Out1 : Outport
  wires:
  Direction Cosine Matrix to Quaternions1/1 -> Demux2/1
  Rotation Matrix to VRML Rotation1/1 -> Out1/1
  Mux2/1 -> Quaternions to Direction Cosine Matrix1/1
  Demux2/4 -> Mux2/3
  Demux2/3 -> Gain4/1
  Gain4/1 -> Mux2/4
  Demux2/1 -> Mux2/1
  Demux2/2 -> Mux2/2
  Quaternions to Direction Cosine Matrix1/1 -> Rotation Matrix to VRML Rotation1/1
  In1/1 -> Direction Cosine Matrix to Quaternions1/1

== system CompleteAttDetSim/Rotation Matrix to VRML 1 ==
  In1 : Inport
  Demux2 : Demux
  Direction Cosine Matrix to Quaternions1 : sharedtransform/Direction Cosine Matrix  to Quaternions  aMode=aMode  action=None  tolerance=eps(2)
      settings: SourceProductName=Aerospace Blockset  SourceProductBaseCode=AE
  Gain4 : Gain  Gain=-1
  Mux2 : Mux
  Quaternions to Direction Cosine Matrix1 : sharedtransform/Quaternions to  Direction Cosine Matrix  aMode=aMode
      settings: SourceProductName=Aerospace Blockset  SourceProductBaseCode=AE
  Rotation Matrix to VRML Rotation1 : vrlib/Utilities/Rotation Matrix to VRML Rotation  maxzero=1e-12
      settings: SourceProductName=Simulink 3D Animation  SourceProductBaseCode=VR
  Out1 : Outport
  wires:
  Direction Cosine Matrix to Quaternions1/1 -> Demux2/1
  Rotation Matrix to VRML Rotation1/1 -> Out1/1
  Mux2/1 -> Quaternions to Direction Cosine Matrix1/1
  Demux2/4 -> Mux2/3
  Demux2/3 -> Gain4/1
  Gain4/1 -> Mux2/4
  Demux2/1 -> Mux2/1
  Demux2/2 -> Mux2/2
  Quaternions to Direction Cosine Matrix1/1 -> Rotation Matrix to VRML Rotation1/1
  In1/1 -> Direction Cosine Matrix to Quaternions1/1

== system CompleteAttDetSim/Sun Sensor ==
  Sun Vector : Inport
  Q ECI2BOD : Inport  Port=2
  Normalize Vector4 : vrlib/Utilities/Normalize Vector  maxzero=0
      settings: SourceProductName=Simulink 3D Animation  SourceProductBaseCode=VR
  Quaternion Rotation : aerolibutil/Quaternion Rotation
  Quaternion Rotation2 : aerolibutil/Quaternion Rotation
  Random Quat Error : MATLAB Function  TreatAsAtomicUnit=on
  Unit Sun Vector BOD : Outport
  wires:
  Sun Vector/1 -> Quaternion Rotation/2
  Random Quat Error/1(quat) -> Quaternion Rotation/1
  Normalize Vector4/1 -> Unit Sun Vector BOD/1
  Q ECI2BOD/1 -> Quaternion Rotation2/1
  Quaternion Rotation2/1 -> Normalize Vector4/1
  Quaternion Rotation/1 -> Quaternion Rotation2/2

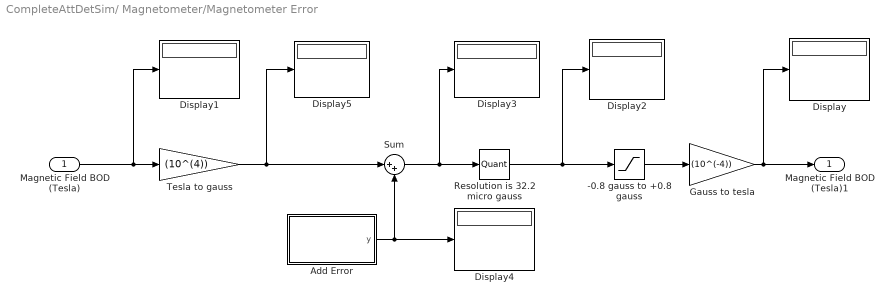
== system CompleteAttDetSim/ Magnetometer/Magnetometer Error ==
  Magnetic Field BOD (Tesla) : Inport
  -0.8 gauss to +0.8 gauss : Saturate  UpperLimit=0.8  LowerLimit=-0.8
  Add Error : MATLAB Function  TreatAsAtomicUnit=on
  Display{,1..5} (6 alike) : Display
  Gauss to tesla : Gain  Gain=(10^(-4))
  Resolution is 32.2 micro gauss : Quantizer  QuantizationInterval=0.0322
  Sum : Sum  Inputs=|++
  Tesla to gauss : Gain  Gain=(10^(4))
  "Magnetic Field BOD (Tesla)1 " : Outport
  wires:
  -0.8 gauss to +0.8 gauss/1 -> Gauss to tesla/1
  Sum/1 -> Display3/1, Resolution is 32.2 micro gauss/1
  Tesla to gauss/1 -> Sum/1, Display5/1
  Add Error/1(y) -> Display4/1, Sum/2
  Magnetic Field BOD (Tesla)/1 -> Display1/1, Tesla to gauss/1
  Gauss to tesla/1 -> "Magnetic Field BOD (Tesla)1 "/1, Display/1
  Resolution is 32.2 micro gauss/1 -> -0.8 gauss to +0.8 gauss/1, Display2/1

== system CompleteAttDetSim/Earth Rotation/Subsystem1 ==
  we : Inport
  Clock : Inport  Port=2
  Display : Display
  MATLAB Function : MATLAB Function  TreatAsAtomicUnit=on
  Product1 : Product
  Earth Rotation Matrix : Outport
  wires:
  Clock/1 -> Product1/2
  we/1 -> Product1/1
  Product1/1 -> MATLAB Function/1(u), Display/1  "fi_earth"
  MATLAB Function/1(y) -> Earth Rotation Matrix/1

== matlab function CompleteAttDetSim/Earth Rotation/Subsystem1/MATLAB Function ==
  data: u input; y output
function y = fcn(u)
y =rotz(u);

== matlab function CompleteAttDetSim/Orbit Propagator/d params ==
  data: grav_parameter input; d_RAAN output; J2 input; earthRadius input; eccentricity input; sm_axis input; inclination input; d_omeg output
function [d_RAAN, d_omeg]=dparams(grav_parameter,J2, earthRadius,eccentricity,sm_axis,inclination)
d_RAAN = -(1.5*J2*grav_parameter^0.5*earthRadius^2/((1-eccentricity^2)*sm_axis^3.5))*cosd(inclination)*180/pi;
d_omeg = d_RAAN*(2.5*sind(inclination)^2 - 2)/cosd(inclination);
end

== matlab function CompleteAttDetSim/Model Attitude Matrix 1/Rotate about x1 ==
  data: u input; y output
function y = fcn(u)
y =rotx(u);

== matlab function CompleteAttDetSim/Orbit Propagator/MATLAB Function ==
  data: avg_anomaly input; eccentricity input; E output; eps input
function E = keplerEq(avg_anomaly,eccentricity,eps)
En  = avg_anomaly;
Ens = En - (En-eccentricity*sin(En)- avg_anomaly)/...
    (1 - eccentricity*cos(En));
while ( abs(Ens-En) > eps )
    En = Ens;
    Ens = En - (En - eccentricity*sin(En) - avg_anomaly)/...
        (1 - eccentricity*cos(En));
end
E = Ens;
end

== matlab function CompleteAttDetSim/Orbit Propagator/Update theta ==
  data: E input; theta output; eccentricity input
function theta = updateTheta(E,eccentricity)
theta=2*atan(tan(E/2)*((1+eccentricity)/(1-eccentricity))^0.5)*180/pi;
end

== matlab function CompleteAttDetSim/Orbit Propagator/Orbital to State ==
  data: orbitalElemets input; Pos output size=[1 3]; Vel output size=[1 3]
function [Pos, Vel] = Orbital2State(orbitalElemets)

% ˜˜˜˜˜˜˜˜˜˜˜˜˜˜˜˜˜˜˜˜˜˜˜˜˜˜˜˜˜˜˜˜˜˜
% This function computes the state vector (r,v) from the
% classical orbital elements (coe).
%
% 
% incl = inclination of the orbit (rad)
% w = argument of perigee (rad)
% TA = true anomaly (rad)
% R3_w - Rotation matrix about the z-axis through the angle w
% R1_i - Rotation matrix about the x-axis through the angle i
% Rot_z - Rotation matrix about the z-axis through the angle RA
% Q_pX - Matrix of the transformation from perifocal to
% geocentric equatorial frame

% r - position vector in the geocentric equatorial frame
% (km)
% v - velocity vector in the geocentric equatorial frame
% (km/s)
%
% User M-functions required: none
% ------------------------------------------------------------
grav_parameter = 398600; 
angMomentum = orbitalElemets(1);
eccentricity = orbitalElemets(2);
RAAN = orbitalElemets(3)*pi/180;
inclination = orbitalElemets(4)*pi/180;
omega = orbitalElemets(5)*pi/180;
theta = orbitalElemets(6)*pi/180;

%perifocal_frame_posVect - position vector in the perifocal frame in kilometers
% perifocal_frame_velVect - velocity vector in the perifocal frame in kilometers per second
perifocal_frame_posVect =(angMomentum^2/grav_parameter)*(1/(1+eccentricity*cos(theta)))*(cos(theta)*[1;0;0]+ sin(theta)*[0;1;0]);
perifocal_frame_velVect =(grav_parameter/angMomentum)*(-sin(theta)*[1;0;0]+(eccentricity+cos(theta))*[0;1;0]);

%Rotation matrix about z-axis through angle RAAN
Rot_zw = [ cos(RAAN) sin(RAAN) 0; -sin(RAAN) cos(RAAN) 0; 0 0 1];
%Rotation matrix about x-axis through the angle of inclination
Rot_xi = [1 0 0; 0 cos(inclination) sin(inclination); 0 -sin(inclination) cos(inclination)];
%Rotation matrix about the z-axis through the angle omega
R3_w = [ cos(omega) sin(omega) 0; -sin(omega) cos(omega) 0; 0 0 1];
%transformation from perifocal to geocentric equatorial frame
Geo_to_equatorial = Rot_zw'*Rot_xi'*R3_w';
% position and velocity vector in the geocentric equatorial frame in kilometers per second
pos = Geo_to_equatorial*perifocal_frame_posVect;
vel = Geo_to_equatorial*perifocal_frame_velVect;

Pos = pos';
Vel = vel';
% ˜˜˜˜˜˜˜˜˜˜˜˜˜˜˜˜˜˜˜˜˜˜˜˜˜˜˜˜˜˜˜˜˜˜˜˜˜˜˜˜˜˜˜˜˜˜˜˜˜˜˜˜˜˜˜˜˜˜˜˜

== matlab function CompleteAttDetSim/IGRF/Convert Local  Spherical to ECI ==
  data: Brad input; Bx output; Btheat input; Bphi input; lat input; LocalSiderealTime input; By output; Bz output
function [Bx,By,Bz] = msph2inert(Brad,Btheat,Bphi,lat, LocalSiderealTime)
lat=lat*pi/180; LocalSiderealTime=LocalSiderealTime*pi/180;
% Coordinate transformation
Bx = (Brad*cos(lat)+Btheat*sin(lat))*cos(LocalSiderealTime) - Bphi*sin(LocalSiderealTime);
By = (Brad*cos(lat)+Btheat*sin(lat))*sin(LocalSiderealTime) + Bphi*cos(LocalSiderealTime);
Bz = (Brad*sin(lat)+Btheat*cos(lat));

== matlab function CompleteAttDetSim/IGRF/ECI2ECEF ==
  data: rECI input; rECEF output; year input; month input; day input; hour input; min input; s input; simtime input
function rECEF=rECI2ECEF(rECI, year, month, day, hour, min, s, simtime )
d2000=367*year-floor((7*(year+(floor(month+9)/12)))/4)+floor(275*month/9)+((hour+(min/60)+((s+simtime)/3600))/24)+day-730531.5;
theta=280.46061837+360.98564736628*d2000;

trans_mat=[cosd(theta) sind(theta) 0; -sind(theta) cosd(theta) 0; 0 0 1];

rECEF=trans_mat*rECI;

end

== matlab function CompleteAttDetSim/IGRF/Local Sidereal Time ==
  data: datevec input; LST output; long input

function LST = locst(datevec,long)
yr=datevec(1); mon=datevec(2); day=datevec(3); hr=datevec(4); min=datevec(5); sec=datevec(6);
UT=( (sec/60.0 + min ) / 60.0 + hr );
J0 = 367.0 * yr  ...
- floor( (7 * (yr + floor( (mon + 9) / 12.0) ) ) * 0.25 )   ...
+ floor( 275 * mon / 9.0 ) ...
+ day + 1721013.5;
JD=J0+(UT/24);
JC = (J0 - 2451545.0)/36525;
GST0 = 100.4606184 + 36000.77004*JC + 0.000387933*JC^2 - 2.583e-8*JC^3; %[deg]
GST0 = mod(GST0, 360);  % GST0 range [0..360]
GST = GST0 + 360.98564724*UT/24;
GST = mod(GST, 360);  % GST0 range [0..360]
LST = GST + long;
LST = mod(LST, 360);  % LST range [0..360]
